simulink model "w2p4"  (R2020a)
settings: Solver=VariableStepAuto  StartTime=0.0  StopTime=10.0  RelTol=1e-3
values from neighbouring files (symbols this model uses):
  b = 3.5077e-06    [w2p4.mat]
  J = 3.2284e-06    [w2p4.mat]
  kd = 120    [w2p4.mat]
  Ke = 0.0274    [w2p4.mat]
  ki = 200    [w2p4.mat]
  kp = 350    [w2p4.mat]
  Kt = 0.0274    [w2p4.mat]
  L = 2.75e-06    [w2p4.mat]
  R = 4    [w2p4.mat]
undefined symbols (not defined in the file or in its folder): N
settings Model: Creator=Shubham  LastModifiedBy=Shubham

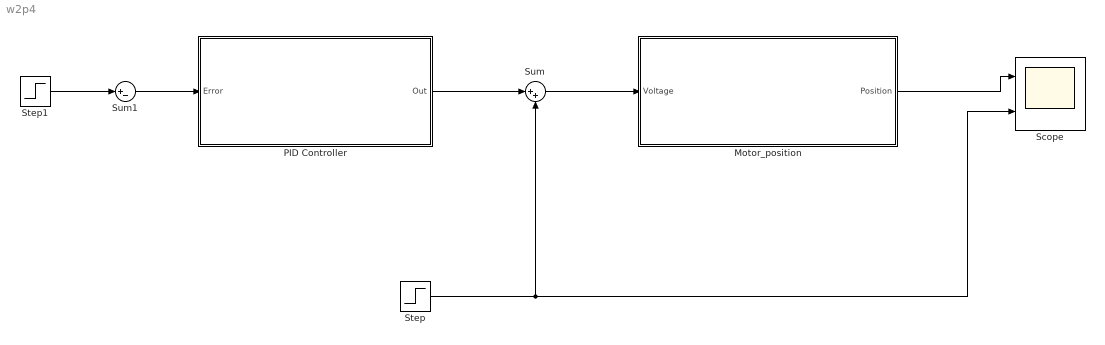
== system w2p4 ==
  Motor_position : Subsystem
  PID Controller : Subsystem
  Scope : Scope  NumInputPorts=2
  Step : Step  SampleTime=0
  Step1 : Step  SampleTime=0
  Sum : Sum  Inputs=|++
  Sum1 : Sum  Inputs=|+-
  wires:
  PID Controller/1(Out) -> Sum/1
  Sum/1 -> Motor_position/1(Voltage)
  Motor_position/1(Position) -> Scope/1
  Step/1 -> Sum/2, Scope/2
  Step1/1 -> Sum1/1
  Sum1/1 -> PID Controller/1(Error)

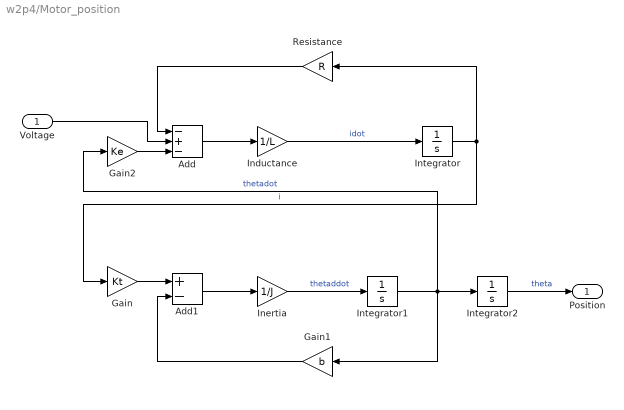
== system w2p4/Motor_position ==
  Voltage : Inport
  Add : Sum  Inputs=-+-
  Add1 : Sum  Inputs=+-
  Gain : Gain  Gain=Kt
  Gain1 : Gain  Gain=b
  Gain2 : Gain  Gain=Ke
  Inductance : Gain  Gain=1/L
  Inertia : Gain  Gain=1/J
  Integrator : Integrator
  Integrator1 : Integrator
  Integrator2 : Integrator
  Resistance : Gain  Gain=R
  Position : Outport
  wires:
  Integrator1/1 -> Gain2/1, Gain1/1, Integrator2/1  "thetadot"
  Inertia/1 -> Integrator1/1  "thetaddot"
  Inductance/1 -> Integrator/1  "idot"
  Integrator/1 -> Gain/1, Resistance/1  "i"
  Integrator2/1 -> Position/1  "theta"
  Add1/1 -> Inertia/1
  Add/1 -> Inductance/1
  Gain/1 -> Add1/1
  Gain1/1 -> Add1/2
  Gain2/1 -> Add/3
  Resistance/1 -> Add/1
  Voltage/1 -> Add/2

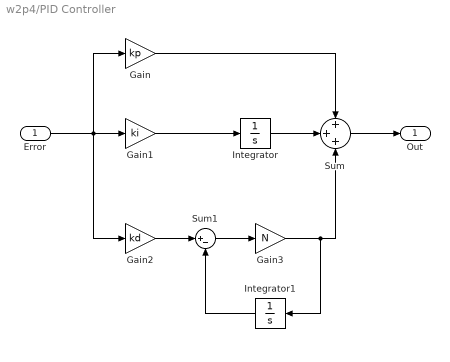
== system w2p4/PID Controller ==
  Error : Inport
  Gain : Gain  Gain=kp
  Gain1 : Gain  Gain=ki
  Gain2 : Gain  Gain=kd
  Gain3 : Gain  Gain=N
  Integrator : Integrator
  Integrator1 : Integrator
  Sum : Sum  Inputs=+++
  Sum1 : Sum  Inputs=|+-
  Out : Outport
  wires:
  Sum/1 -> Out/1
  Gain1/1 -> Integrator/1
  Integrator/1 -> Sum/2
  Gain/1 -> Sum/1
  Sum1/1 -> Gain3/1
  Gain2/1 -> Sum1/1
  Integrator1/1 -> Sum1/2
  Gain3/1 -> Integrator1/1, Sum/3
  Error/1 -> Gain2/1, Gain/1, Gain1/1
